simulink model "seminar4_topic2_2"  (R2019b)
settings: Solver=VariableStepAuto  StartTime=0.0  StopTime=0.01  RelTol=1e-3
model workspace (MAT data in the model file):
  d = 50
  s = 50
  s2 = 50
values from neighbouring files (symbols this model uses):
  tem1 = d    [analysis2.m]
  tem2 = d    [analysis2.m]
libraries: powerlib x21, powerlib_meascontrol x1
settings Model: Creator=96547  LastModifiedBy=96547
settings DataIOCC: ReturnWorkspaceOutputs=off

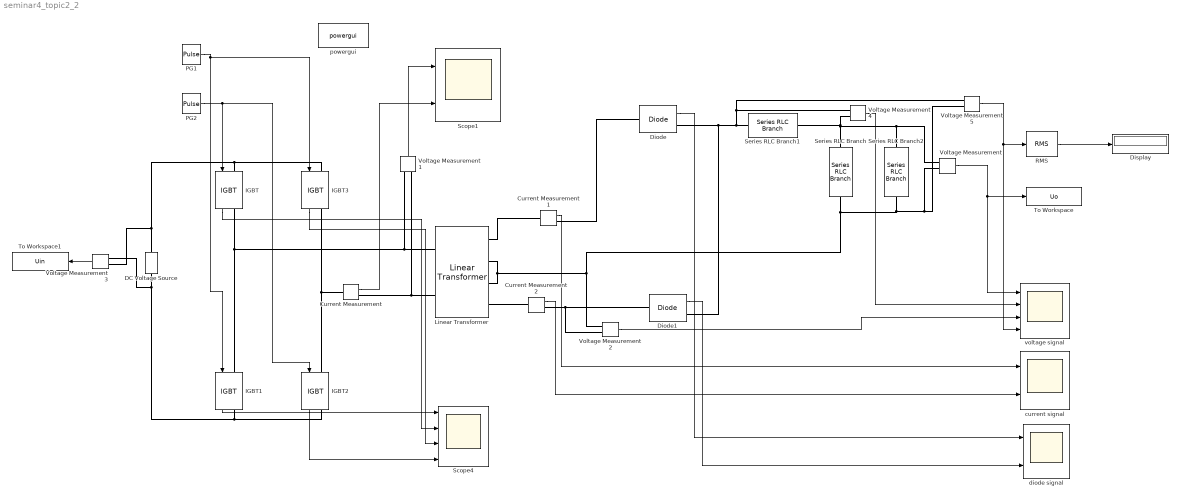
== system seminar4_topic2_2 ==
  Current Measurement : powerlib/Measurements/Current Measurement  PhasorSimulation=off  OutputType=Complex  PSBequivalent=0
      settings: SourceProductName=Simscape Electrical
  Current Measurement1 : powerlib/Measurements/Current Measurement  PhasorSimulation=off  OutputType=Complex  PSBequivalent=0
      settings: SourceProductName=Simscape Electrical
  Current Measurement2 : powerlib/Measurements/Current Measurement  PhasorSimulation=off  OutputType=Complex  PSBequivalent=0
      settings: SourceProductName=Simscape Electrical
  DC Voltage Source : powerlib/Electrical Sources/DC Voltage Source  Amplitude=600  Measurements=None
      settings: SourceProductName=Simscape Electrical
  Diode : powerlib/Power Electronics/Diode  Ron=0  Lon=0  Vf=0.8  IC=0  UseSnubber=0  Rs=500  Cs=250e-9  Measurements=on
      settings: SourceProductName=Simscape Electrical
  Diode1 : powerlib/Power Electronics/Diode  Ron=0  Lon=0  Vf=0.8  IC=0  UseSnubber=0  Rs=500  Cs=250e-9  Measurements=on
      settings: SourceProductName=Simscape Electrical
  Display : Display
  IGBT{,1..3} (4 alike) : powerlib/Power Electronics/IGBT  Ron=0.001  Lon=0  Vf=1  Tf=1e-6  Tt=2e-6  IC=0  Rs=1e5  Cs=inf  Measurements=on
      settings: SourceProductName=Simscape Electrical
  Linear Transformer : powerlib/Elements/Linear Transformer  UNITS=pu  NominalPower=[ 250e6 100000 ]  winding1="[ 1260e3  0 0 ]"  winding2="[ 315e3  0 0 ]"  ThreeWindings=on  winding3=[ 315e3 0 0 ]  RmLm=[ 500 500 ]  Measurements=None  DataType=off
      settings: SourceProductName=Simscape Electrical
  PG1 : DiscretePulseGenerator  PulseType=Time based  Period=1e-5  PulseWidth=tem1
  PG2 : DiscretePulseGenerator  PulseType=Time based  Period=1e-5  PulseWidth=tem2  PhaseDelay=0.5e-5
  RMS : powerlib_meascontrol/Measurements/RMS  TrueRMS=on  Freq=1e5  RMSInit=0  Ts=0
      settings: SourceProductName=Simscape Electrical
  Scope1 : Scope  NumInputPorts=2
  Scope4 : Scope  NumInputPorts=4
  Series RLC Branch : powerlib/Elements/Series RLC Branch  LConnTagsString=__new0  RConnTagsString=__new0  BranchType=C  Resistance=1  Inductance=1e-3  SetiL0=off  InitialCurrent=0  Capacitance=200e-6  Setx0=off  InitialVoltage=0  Measurements=None
      settings: SourceProductName=Simscape Electrical
  Series RLC Branch1 : powerlib/Elements/Series RLC Branch  LConnTagsString=__new0  RConnTagsString=__new0  BranchType=L  Resistance=1  Inductance=300e-6  SetiL0=off  InitialCurrent=0  Capacitance=1e-6  Setx0=off  InitialVoltage=0  Measurements=None
      settings: SourceProductName=Simscape Electrical
  Series RLC Branch2 : powerlib/Elements/Series RLC Branch  LConnTagsString=__new0  RConnTagsString=__new0  BranchType=R  Resistance=10  Inductance=1e-3  SetiL0=off  InitialCurrent=0  Capacitance=1e-6  Setx0=off  InitialVoltage=0  Measurements=None
      settings: SourceProductName=Simscape Electrical
  To Workspace : ToWorkspace  VariableName=Uo  SampleTime=-1
      settings: Save2DSignal=2-D array (concatenate along first dimension)
  To Workspace1 : ToWorkspace  VariableName=Uin  SampleTime=-1
      settings: Save2DSignal=2-D array (concatenate along first dimension)
  Voltage Measurement{,1..5} (6 alike) : powerlib/Measurements/Voltage Measurement  PhasorSimulation=off  OutputType=Complex  PSBequivalent=0
      settings: SourceProductName=Simscape Electrical
  current signal : Scope  NumInputPorts=2
  diode signal : Scope  NumInputPorts=2
  powergui : powerlib/powergui  Priority=1  SimulationMode=Continuous  SampleTime=50e-6  frequency=60  Iterations=50  frequencyindice=0  Pbase=100e6  ErrMax=1e-4  UnitsV=kV  UnitsW=MW  buscounter=0  FunctionMessages=off  echomessages=off  EnableUseOfTLC=off  CurrentSourceSwitches=off  DisableSnubberDevices=off  DisableRonSwitches=off  DisableVfSwitches=off  DisplayEquations=off  AutomaticDiscreteSolvers=off  SolverType=Tustin/Backward Euler (TBE)  Interpol=off  ExternalGateDelay=off  methode=off  Ts=100  x0status=blocks  SPID=on  SwTol=0  HookPort=off  NonlinearTolerance=1e-4  nMaxIteration=100  ContinueOnMaxIteration=off  RestoreLinks=warning  ResistiveCurrentMeasurement=off  Frange=[0:2:500]  Ylog=off  Xlog=on  ShowGrid=off  save=off  variable=ZData  structure=0  ZoomFFT=off  StartTime=0.0  cycles=1  DisplayStyle=1  fundamental=60  FreqAxis=off  MaxFrequency=1000  frequencyindicesteady=1  RmsSteady=1  display=off
      settings: SourceProductName=Simscape Electrical
  voltage signal : Scope  NumInputPorts=4
  wires:
  PG2/1 -> IGBT2/1, IGBT/1
  PG1/1 -> IGBT1/1, IGBT3/1
  Current Measurement/1 -> Scope1/2
  Voltage Measurement1/1 -> Scope1/1
  Current Measurement1/1 -> current signal/1
  Current Measurement2/1 -> current signal/2
  Voltage Measurement2/1 -> voltage signal/3
  Voltage Measurement/1 -> To Workspace/1, voltage signal/1
  RMS/1 -> Display/1
  Diode/1 -> diode signal/1
  Diode1/1 -> diode signal/2
  IGBT1/1 -> Scope4/1
  IGBT/1 -> Scope4/2
  IGBT3/1 -> Scope4/3
  IGBT2/1 -> Scope4/4
  Voltage Measurement3/1 -> To Workspace1/1
  Voltage Measurement4/1 -> voltage signal/2
  Voltage Measurement5/1 -> voltage signal/4, RMS/1
  connections:
  IGBT3/RConn1 -- Current Measurement/LConn1 -- IGBT2/LConn1
  IGBT/RConn1 -- Voltage Measurement1/LConn1 -- Linear Transformer/LConn1 -- IGBT1/LConn1
  DC Voltage Source/RConn1 -- Voltage Measurement3/LConn1 -- IGBT3/LConn1 -- IGBT/LConn1
  DC Voltage Source/LConn1 -- Voltage Measurement3/LConn2 -- IGBT2/RConn1 -- IGBT1/RConn1
  Linear Transformer/RConn2 -- Series RLC Branch/RConn1 -- Voltage Measurement5/LConn2 -- Voltage Measurement/LConn2 -- Series RLC Branch2/RConn1 -- Voltage Measurement2/LConn1 -- Linear Transformer/RConn3
  Series RLC Branch1/LConn1 -- Voltage Measurement5/LConn1 -- Voltage Measurement4/LConn1 -- Diode1/RConn1 -- Diode/RConn1
  Series RLC Branch1/RConn1 -- Series RLC Branch2/LConn1 -- Voltage Measurement/LConn1 -- Series RLC Branch/LConn1 -- Voltage Measurement4/LConn2
  Current Measurement/RConn1 -- Voltage Measurement1/LConn2 -- Linear Transformer/LConn2
  Linear Transformer/RConn1 -- Current Measurement1/LConn1
  Current Measurement1/RConn1 -- Diode/LConn1
  Diode1/LConn1 -- Voltage Measurement2/LConn2 -- Current Measurement2/RConn1
  Current Measurement2/LConn1 -- Linear Transformer/RConn4
